simulink subsystem "Controlador_BC"  (R2024b)
settings: Solver=VariableStepAuto  StartTime=0.0  StopTime=10.0  RelTol=1e-3
settings Model: Creator=Chenfu  LastModifiedBy=Chenfu

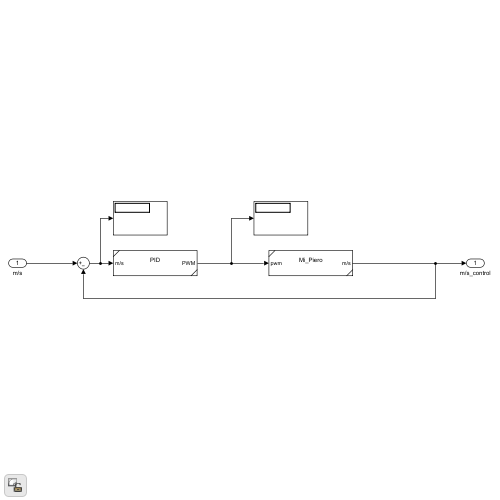
[thumbnail: Simulink's stored preview of the top-level diagram]
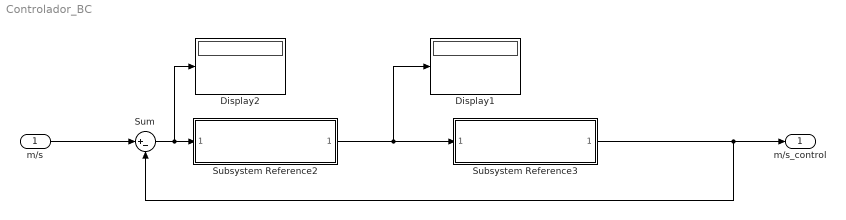
== system Controlador_BC ==
  m/s : Inport
  Display1 : Display
  Display2 : Display
  Subsystem Reference2 : Subsystem  ReferencedSubsystem=PID
  Subsystem Reference3 : Subsystem  ReferencedSubsystem=Mi_Piero
  Sum : Sum  Inputs=|+-
  m/s_control : Outport
  wires:
  Sum/1 -> Display2/1, Subsystem Reference2/1
  Subsystem Reference2/1 -> Display1/1, Subsystem Reference3/1
  Subsystem Reference3/1 -> m/s_control/1, Sum/2
  m/s/1 -> Sum/1
